simulink model "A1Requirements"  (R2022b)
settings: Solver=VariableStepAuto  StartTime=0.0  StopTime=10.0  RelTol=1e-3
settings Model: Creator=coler  LastModifiedBy=TheCoaler

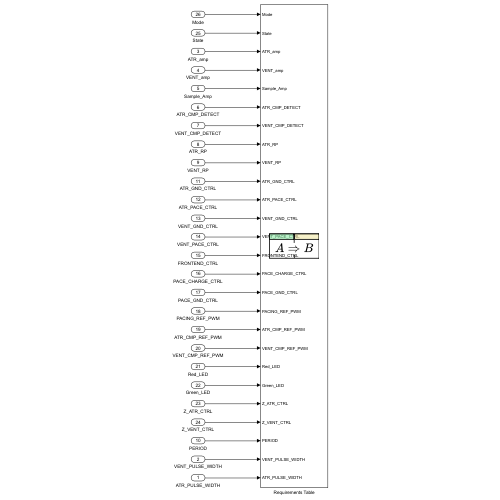
[thumbnail: Simulink's stored preview of the top-level diagram]
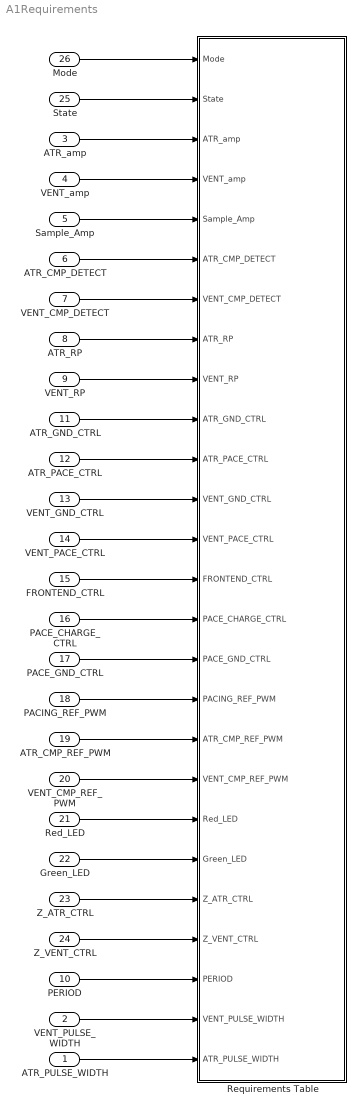
== system A1Requirements ==
  ATR_PULSE_WIDTH : Inport  OutDataTypeStr=int32
  VENT_PULSE_WIDTH : Inport  Port=2
  ATR_amp : Inport  Port=3
  VENT_amp : Inport  Port=4
  Sample_Amp : Inport  Port=5
  ATR_CMP_DETECT : Inport  Port=6
  VENT_CMP_DETECT : Inport  Port=7
  ATR_RP : Inport  Port=8
  VENT_RP : Inport  Port=9
  PERIOD : Inport  Port=10
  ATR_GND_CTRL : Inport  Port=11  OutDataTypeStr=int32
  ATR_PACE_CTRL : Inport  Port=12  OutDataTypeStr=int32
  VENT_GND_CTRL : Inport  Port=13  OutDataTypeStr=int32
  VENT_PACE_CTRL : Inport  Port=14  OutDataTypeStr=int32
  FRONTEND_CTRL : Inport  Port=15  OutDataTypeStr=int32
  PACE_CHARGE_CTRL : Inport  Port=16  OutDataTypeStr=int32
  PACE_GND_CTRL : Inport  Port=17  OutDataTypeStr=int32
  PACING_REF_PWM : Inport  Port=18  OutDataTypeStr=int32
  ATR_CMP_REF_PWM : Inport  Port=19  OutDataTypeStr=int32
  VENT_CMP_REF_PWM : Inport  Port=20  OutDataTypeStr=int32
  Red_LED : Inport  Port=21  OutDataTypeStr=int32
  Green_LED : Inport  Port=22  OutDataTypeStr=int32
  Z_ATR_CTRL : Inport  Port=23  OutDataTypeStr=int32
  Z_VENT_CTRL : Inport  Port=24  OutDataTypeStr=int32
  State : Inport  Port=25  OutDataTypeStr=int32
  Mode : Inport  Port=26  OutDataTypeStr=int32
  Requirements Table : Requirements Table  TreatAsAtomicUnit=on
  wires:
  ATR_PULSE_WIDTH/1 -> Requirements Table/26(ATR_PULSE_WIDTH)
  VENT_PULSE_WIDTH/1 -> Requirements Table/25(VENT_PULSE_WIDTH)
  ATR_amp/1 -> Requirements Table/3(ATR_amp)
  VENT_amp/1 -> Requirements Table/4(VENT_amp)
  Sample_Amp/1 -> Requirements Table/5(Sample_Amp)
  ATR_CMP_DETECT/1 -> Requirements Table/6(ATR_CMP_DETECT)
  VENT_CMP_DETECT/1 -> Requirements Table/7(VENT_CMP_DETECT)
  ATR_RP/1 -> Requirements Table/8(ATR_RP)
  VENT_RP/1 -> Requirements Table/9(VENT_RP)
  PERIOD/1 -> Requirements Table/24(PERIOD)
  ATR_GND_CTRL/1 -> Requirements Table/10(ATR_GND_CTRL)
  ATR_PACE_CTRL/1 -> Requirements Table/11(ATR_PACE_CTRL)
  VENT_GND_CTRL/1 -> Requirements Table/12(VENT_GND_CTRL)
  VENT_PACE_CTRL/1 -> Requirements Table/13(VENT_PACE_CTRL)
  FRONTEND_CTRL/1 -> Requirements Table/14(FRONTEND_CTRL)
  PACE_CHARGE_CTRL/1 -> Requirements Table/15(PACE_CHARGE_CTRL)
  PACE_GND_CTRL/1 -> Requirements Table/16(PACE_GND_CTRL)
  PACING_REF_PWM/1 -> Requirements Table/17(PACING_REF_PWM)
  ATR_CMP_REF_PWM/1 -> Requirements Table/18(ATR_CMP_REF_PWM)
  VENT_CMP_REF_PWM/1 -> Requirements Table/19(VENT_CMP_REF_PWM)
  Red_LED/1 -> Requirements Table/20(Red_LED)
  Green_LED/1 -> Requirements Table/21(Green_LED)
  Z_ATR_CTRL/1 -> Requirements Table/22(Z_ATR_CTRL)
  Z_VENT_CTRL/1 -> Requirements Table/23(Z_VENT_CTRL)
  State/1 -> Requirements Table/2(State)
  Mode/1 -> Requirements Table/1(Mode)

== stateflow chart A1Requirements/Requirements Table ==
  (default) -> (junction 1073744062)
  (junction 1073744062) -> (junction 1073744063) : {
      | % SF_REQ_REV_07
      | }
  (junction 1073744063) -> (junction 1073744065) : {
      | % HEADER_ASSIGNMENTS
      |
      | }
  (junction 1073744065) -> (junction 1073744067) : {
      | % START_A_4
      | }
  (junction 1073744067) -> (junction 1073744069) : {
      | }
  (junction 1073744069) -> (junction 1073744071)
  (junction 1073744071) -> (junction 1073744073) : {
      | }
  (junction 1073744073) -> (junction 1073744075) : {
      | % END_A_4
      | }
  (junction 1073744075) -> (junction 1073744077) : {
      | % START_R_1
      | }
  (junction 1073744077) -> (junction 1073744079) : {
      | }
  (junction 1073744079) -> (junction 1073744081)
  (junction 1073744081) -> (junction 1073744083) [order 1] : [((~((prev(PACE_CHARGE_CTRL)) == (0))))]
  (junction 1073744081) -> (junction 1073744089) [order 2]
  (junction 1073744083) -> (junction 1073744085) : {
      | reqtable_postcondition((((ATR_PACE_CTRL) == (0))) && (((VENT_PACE_CTRL) == (0))) && (((PACING_REF_PWM) >= (0) && (PACING_REF_PWM) <= (5))), 'R:1');
      |
      |
      | }
  (junction 1073744085) -> (junction 1073744087) : {
      | }
  (junction 1073744087) -> (junction 1073744089)
  (junction 1073744089) -> (junction 1073744091)
  (junction 1073744091) -> (junction 1073744093) : {
      | % END_R_1
      | }
  (junction 1073744093) -> (junction 1073744095) : {
      | % START_R_7
      | }
  (junction 1073744095) -> (junction 1073744097) : {
      | }
  (junction 1073744097) -> (junction 1073744099)
  (junction 1073744099) -> (junction 1073744101) [order 1] : [((~((prev(ATR_PACE_CTRL)) == (0)))) && ((~((prev(VENT_PACE_CTRL)) == (0))))]
  (junction 1073744099) -> (junction 1073744107) [order 2]
  (junction 1073744101) -> (junction 1073744103) : {
      | reqtable_postcondition((((PACE_CHARGE_CTRL) == (0))), 'R:2');
      |
      |
      | }
  (junction 1073744103) -> (junction 1073744105) : {
      | }
  (junction 1073744105) -> (junction 1073744107)
  (junction 1073744107) -> (junction 1073744109)
  (junction 1073744109) -> (junction 1073744111) : {
      | % END_R_7
      | }
  (junction 1073744111) -> (junction 1073744113) : {
      | % START_R_58
      | }
  (junction 1073744113) -> (junction 1073744115) : {
      | }
  (junction 1073744115) -> (junction 1073744117)
  (junction 1073744117) -> (junction 1073744119) [order 1] : [(((ATR_CMP_DETECT) == (1)))]
  (junction 1073744117) -> (junction 1073744125) [order 2]
  (junction 1073744119) -> (junction 1073744121) : {
      | reqtable_postcondition((((ATR_CMP_REF_PWM) > (5))), 'R:3');
      |
      |
      | }
  (junction 1073744121) -> (junction 1073744123) : {
      | }
  (junction 1073744123) -> (junction 1073744125)
  (junction 1073744125) -> (junction 1073744127)
  (junction 1073744127) -> (junction 1073744129) : {
      | % END_R_58
      | }
  (junction 1073744129) -> (junction 1073744131) : {
      | % START_R_64
      | }
  (junction 1073744131) -> (junction 1073744133) : {
      | }
  (junction 1073744133) -> (junction 1073744135)
  (junction 1073744135) -> (junction 1073744137) [order 1] : [(((ATR_CMP_DETECT) == (0)))]
  (junction 1073744135) -> (junction 1073744143) [order 2]
  (junction 1073744137) -> (junction 1073744139) : {
      | reqtable_postcondition((((ATR_CMP_REF_PWM) < (5))), 'R:4');
      |
      |
      | }
  (junction 1073744139) -> (junction 1073744141) : {
      | }
  (junction 1073744141) -> (junction 1073744143)
  (junction 1073744143) -> (junction 1073744145)
  (junction 1073744145) -> (junction 1073744147) : {
      | % END_R_64
      | }
  (junction 1073744147) -> (junction 1073744149) : {
      | % START_R_61
      | }
  (junction 1073744149) -> (junction 1073744151) : {
      | }
  (junction 1073744151) -> (junction 1073744153)
  (junction 1073744153) -> (junction 1073744155) [order 1] : [(((VENT_CMP_DETECT) == (1)))]
  (junction 1073744153) -> (junction 1073744161) [order 2]
  (junction 1073744155) -> (junction 1073744157) : {
      | reqtable_postcondition((((VENT_CMP_REF_PWM) > (5))), 'R:5');
      |
      |
      | }
  (junction 1073744157) -> (junction 1073744159) : {
      | }
  (junction 1073744159) -> (junction 1073744161)
  (junction 1073744161) -> (junction 1073744163)
  (junction 1073744163) -> (junction 1073744165) : {
      | % END_R_61
      | }
  (junction 1073744165) -> (junction 1073744167) : {
      | % START_R_67
      | }
  (junction 1073744167) -> (junction 1073744169) : {
      | }
  (junction 1073744169) -> (junction 1073744171)
  (junction 1073744171) -> (junction 1073744173) [order 1] : [(((VENT_CMP_DETECT) == (0)))]
  (junction 1073744171) -> (junction 1073744179) [order 2]
  (junction 1073744173) -> (junction 1073744175) : {
      | reqtable_postcondition((((VENT_CMP_REF_PWM) < (5))), 'R:6');
      |
      |
      | }
  (junction 1073744175) -> (junction 1073744177) : {
      | }
  (junction 1073744177) -> (junction 1073744179)
  (junction 1073744179) -> (junction 1073744181)
  (junction 1073744181) -> (junction 1073744183) : {
      | % END_R_67
      | }
  (junction 1073744183) -> (junction 1073744185) : {
      | % START_R_46
      | }
  (junction 1073744185) -> (junction 1073744187) : {
      | }
  (junction 1073744187) -> (junction 1073744189) : {
      |
      |
      | }
  (junction 1073744189) -> (junction 1073744191) : {
      | }
  (junction 1073744191) -> (junction 1073744193) : {
      | % START_R_52
      | }
  (junction 1073744193) -> (junction 1073744195) : {
      | }
  (junction 1073744195) -> (junction 1073744197)
  (junction 1073744197) -> (junction 1073744199) [order 1] : [(((Mode) == (1))) && (((State) == (1)))]
  (junction 1073744197) -> (junction 1073744205) [order 2]
  (junction 1073744199) -> (junction 1073744201) : {
      | reqtable_postcondition((((ATR_PACE_CTRL) == (0))) && (((VENT_PACE_CTRL) == (0))) && (((PACE_GND_CTRL) == (1))) && (((Z_ATR_CTRL) == (0))) && (((Z_VENT_CTRL) == (0))) && (((ATR_GND_CTRL) == (1))) && (((VENT_GND_CTRL) == (0))) && (((Red_LED) == (0))) && (((PACING_REF_PWM) == (ATR_amp))) && (((PACE_CHARGE_CTRL) == (1))), 'R:7.1');
      |
      |
      | }
  (junction 1073744201) -> (junction 1073744203) : {
      | }
  (junction 1073744203) -> (junction 1073744205)
  (junction 1073744205) -> (junction 1073744207)
  (junction 1073744207) -> (junction 1073744209) : {
      | % END_R_52
      | }
  (junction 1073744209) -> (junction 1073744211) : {
      | % START_R_55
      | }
  (junction 1073744211) -> (junction 1073744213) : {
      | }
  (junction 1073744213) -> (junction 1073744215)
  (junction 1073744215) -> (junction 1073744217) [order 1] : [(((Mode) == (1))) && (((State) == (0)))]
  (junction 1073744215) -> (junction 1073744223) [order 2]
  (junction 1073744217) -> (junction 1073744219) : {
      | reqtable_postcondition((((ATR_PACE_CTRL) == (1))) && (((VENT_PACE_CTRL) == (0))) && (((PACE_GND_CTRL) == (1))) && (((Z_ATR_CTRL) == (0))) && (((Z_VENT_CTRL) == (0))) && (((ATR_GND_CTRL) == (0))) && (((VENT_GND_CTRL) == (0))) && (((Red_LED) == (1))) && (((PACING_REF_PWM) == (ATR_amp))) && (((PACE_CHARGE_CTRL) == (0))), 'R:7.2');
      |
      |
      | }
  (junction 1073744219) -> (junction 1073744221) : {
      | }
  (junction 1073744221) -> (junction 1073744223)
  (junction 1073744223) -> (junction 1073744225)
  (junction 1073744225) -> (junction 1073744227) : {
      | % END_R_55
      | }
  (junction 1073744227) -> (junction 1073744229) : {
      | % END_R_46
      | }
  (junction 1073744229) -> (junction 1073744339) : {
      | % START_R_49
      | }
  (junction 1073744339) -> (junction 1073744341) : {
      | }
  (junction 1073744341) -> (junction 1073744343) : {
      |
      |
      | }
  (junction 1073744343) -> (junction 1073744345) : {
      | }
  (junction 1073744345) -> (junction 1073744441) : {
      | % START_R_76
      | }
  (junction 1073744441) -> (junction 1073744443) : {
      | }
  (junction 1073744443) -> (junction 1073744445)
  (junction 1073744445) -> (junction 1073744447) [order 1] : [(((Mode) == (1))) && (((State) == (1)))]
  (junction 1073744445) -> (junction 1073744453) [order 2]
  (junction 1073744447) -> (junction 1073744449) : {
      | reqtable_postcondition((((ATR_PACE_CTRL) == (0))) && (((VENT_PACE_CTRL) == (0))) && (((PACE_GND_CTRL) == (1))) && (((Z_ATR_CTRL) == (0))) && (((Z_VENT_CTRL) == (0))) && (((ATR_GND_CTRL) == (0))) && (((VENT_GND_CTRL) == (1))) && (((Red_LED) == (0))) && (((PACING_REF_PWM) == (VENT_amp))) && (((PACE_CHARGE_CTRL) == (1))), 'R:8.1');
      |
      |
      | }
  (junction 1073744449) -> (junction 1073744451) : {
      | }
  (junction 1073744451) -> (junction 1073744453)
  (junction 1073744453) -> (junction 1073744455)
  (junction 1073744455) -> (junction 1073744457) : {
      | % END_R_76
      | }
  (junction 1073744457) -> (junction 1073744462) : {
      | % START_R_79
      | }
  (junction 1073744462) -> (junction 1073744464) : {
      | }
  (junction 1073744464) -> (junction 1073744466)
  (junction 1073744466) -> (junction 1073744468) [order 1] : [(((Mode) == (1))) && (((State) == (0)))]
  (junction 1073744466) -> (junction 1073744474) [order 2]
  (junction 1073744468) -> (junction 1073744470) : {
      | reqtable_postcondition((((ATR_PACE_CTRL) == (0))) && (((VENT_PACE_CTRL) == (1))) && (((PACE_GND_CTRL) == (1))) && (((Z_ATR_CTRL) == (0))) && (((Z_VENT_CTRL) == (0))) && (((ATR_GND_CTRL) == (0))) && (((VENT_GND_CTRL) == (0))) && (((Red_LED) == (1))) && (((PACING_REF_PWM) == (VENT_amp))) && (((PACE_CHARGE_CTRL) == (0))), 'R:8.2');
      |
      |
      | }
  (junction 1073744470) -> (junction 1073744472) : {
      | }
  (junction 1073744472) -> (junction 1073744474)
  (junction 1073744474) -> (junction 1073744476)
  (junction 1073744476) -> (junction 1073744478) : {
      | % END_R_79
      | }
  (junction 1073744478) -> (junction 1073744357) : {
      | % END_R_49
      | }
  (junction 1073744357) -> (junction 1073744271) : {
      | % START_R_10
      | }
  (junction 1073744271) -> (junction 1073744273) : {
      | }
  (junction 1073744273) -> (junction 1073744275) : {
      |
      |
      | }
  (junction 1073744275) -> (junction 1073744277) : {
      | }
  (junction 1073744277) -> (junction 1073744483) : {
      | % START_R_70
      | }
  (junction 1073744483) -> (junction 1073744485) : {
      | }
  (junction 1073744485) -> (junction 1073744487)
  (junction 1073744487) -> (junction 1073744489) [order 1] : [(((Mode) == (1))) && (((State) == (1)))]
  (junction 1073744487) -> (junction 1073744495) [order 2]
  (junction 1073744489) -> (junction 1073744491) : {
      | reqtable_postcondition((((ATR_PACE_CTRL) == (0))) && (((VENT_PACE_CTRL) == (0))) && (((PACE_GND_CTRL) == (1))) && (((Z_ATR_CTRL) == (0))) && (((Z_VENT_CTRL) == (0))) && (((ATR_GND_CTRL) == (1))) && (((VENT_GND_CTRL) == (0))) && (((Red_LED) == (0))) && (((Green_LED) == (1))) && (((PACING_REF_PWM) == (ATR_amp))) && (((PACE_CHARGE_CTRL) == (1))) && (((ATR_CMP_REF_PWM) == (Sample_Amp))) && (((FRONTEND_CTRL) == (1))), 'R:9.1');
      |
      |
      | }
  (junction 1073744491) -> (junction 1073744493) : {
      | }
  (junction 1073744493) -> (junction 1073744495)
  (junction 1073744495) -> (junction 1073744497)
  (junction 1073744497) -> (junction 1073744499) : {
      | % END_R_70
      | }
  (junction 1073744499) -> (junction 1073744504) : {
      | % START_R_73
      | }
  (junction 1073744504) -> (junction 1073744506) : {
      | }
  (junction 1073744506) -> (junction 1073744508)
  (junction 1073744508) -> (junction 1073744510) [order 1] : [(((Mode) == (1))) && (((State) == (0)))]
  (junction 1073744508) -> (junction 1073744516) [order 2]
  (junction 1073744510) -> (junction 1073744512) : {
      | reqtable_postcondition((((ATR_PACE_CTRL) == (1))) && (((VENT_PACE_CTRL) == (0))) && (((PACE_GND_CTRL) == (1))) && (((Z_ATR_CTRL) == (0))) && (((Z_VENT_CTRL) == (0))) && (((ATR_GND_CTRL) == (0))) && (((VENT_GND_CTRL) == (0))) && (((Red_LED) == (1))) && (((PACING_REF_PWM) == (ATR_amp))) && (((PACE_CHARGE_CTRL) == (0))) && (((FRONTEND_CTRL) == (0))), 'R:9.2');
      |
      |
      | }
  (junction 1073744512) -> (junction 1073744514) : {
      | }
  (junction 1073744514) -> (junction 1073744516)
  (junction 1073744516) -> (junction 1073744518)
  (junction 1073744518) -> (junction 1073744520) : {
      | % END_R_73
      | }
  (junction 1073744520) -> (junction 1073744289) : {
      | % END_R_10
      | }
  (junction 1073744289) -> (junction 1073744407) : {
      | % START_R_13
      | }
  (junction 1073744407) -> (junction 1073744409) : {
      | }
  (junction 1073744409) -> (junction 1073744411) : {
      |
      |
      | }
  (junction 1073744411) -> (junction 1073744413) : {
      | }
  (junction 1073744413) -> (junction 1073744525) : {
      | % START_R_82
      | }
  (junction 1073744525) -> (junction 1073744527) : {
      | }
  (junction 1073744527) -> (junction 1073744529)
  (junction 1073744529) -> (junction 1073744531) [order 1] : [(((Mode) == (1))) && (((State) == (1)))]
  (junction 1073744529) -> (junction 1073744537) [order 2]
  (junction 1073744531) -> (junction 1073744533) : {
      | reqtable_postcondition((((ATR_PACE_CTRL) == (0))) && (((VENT_PACE_CTRL) == (0))) && (((PACE_GND_CTRL) == (1))) && (((Z_ATR_CTRL) == (0))) && (((Z_VENT_CTRL) == (0))) && (((ATR_GND_CTRL) == (0))) && (((VENT_GND_CTRL) == (1))) && (((Red_LED) == (0))) && (((Green_LED) == (1))) && (((PACING_REF_PWM) == (VENT_amp))) && (((PACE_CHARGE_CTRL) == (1))) && (((ATR_CMP_REF_PWM) == (Sample_Amp))) && (((FRONTEND_CTRL) == (1))), 'R:10.1');
      |
      |
      | }
  (junction 1073744533) -> (junction 1073744535) : {
      | }
  (junction 1073744535) -> (junction 1073744537)
  (junction 1073744537) -> (junction 1073744539)
  (junction 1073744539) -> (junction 1073744541) : {
      | % END_R_82
      | }
  (junction 1073744541) -> (junction 1073744546) : {
      | % START_R_85
      | }
  (junction 1073744546) -> (junction 1073744548) : {
      | }
  (junction 1073744548) -> (junction 1073744550)
  (junction 1073744550) -> (junction 1073744552) [order 1] : [(((Mode) == (1))) && (((State) == (0)))]
  (junction 1073744550) -> (junction 1073744558) [order 2]
  (junction 1073744552) -> (junction 1073744554) : {
      | reqtable_postcondition((((ATR_PACE_CTRL) == (0))) && (((VENT_PACE_CTRL) == (1))) && (((PACE_GND_CTRL) == (1))) && (((Z_ATR_CTRL) == (0))) && (((Z_VENT_CTRL) == (0))) && (((ATR_GND_CTRL) == (0))) && (((VENT_GND_CTRL) == (0))) && (((Red_LED) == (1))) && (((PACING_REF_PWM) == (VENT_amp))) && (((PACE_CHARGE_CTRL) == (0))) && (((FRONTEND_CTRL) == (0))), 'R:10.2');
      |
      |
      | }
  (junction 1073744554) -> (junction 1073744556) : {
      | }
  (junction 1073744556) -> (junction 1073744558)
  (junction 1073744558) -> (junction 1073744560)
  (junction 1073744560) -> (junction 1073744562) : {
      | % END_R_85
      | }
  (junction 1073744562) -> (junction 1073744425) : {
      | % END_R_13
      | }
  data: Mode input; State input; ATR_amp input; VENT_amp input; Sample_Amp input; ATR_CMP_DETECT input; VENT_CMP_DETECT input; ATR_RP input; VENT_RP input; ATR_GND_CTRL input; ATR_PACE_CTRL input; VENT_GND_CTRL input; VENT_PACE_CTRL input; FRONTEND_CTRL input; PACE_CHARGE_CTRL input; PACE_GND_CTRL input; PACING_REF_PWM input; ATR_CMP_REF_PWM input; VENT_CMP_REF_PWM input; Red_LED input; Green_LED input; Z_ATR_CTRL input; Z_VENT_CTRL input; PERIOD input; VENT_PULSE_WIDTH input; ATR_PULSE_WIDTH input
